simulink model "q3_3_2"  (R2022a)
settings: Solver=FixedStepAuto  StartTime=0.0  StopTime=200.0  FixedStep=5e-3  RelTol=1e-3
settings Model: Creator=user  LastModifiedBy=user

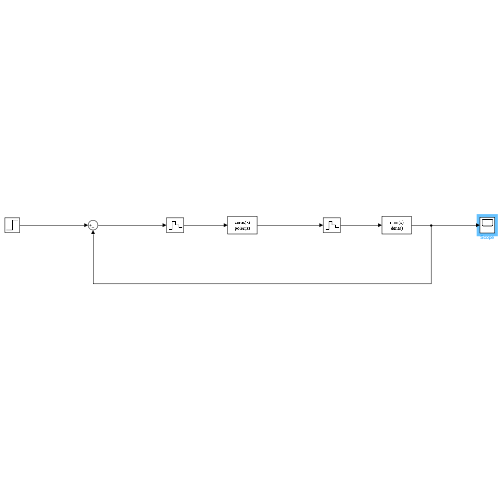
[thumbnail: Simulink's stored preview of the top-level diagram]
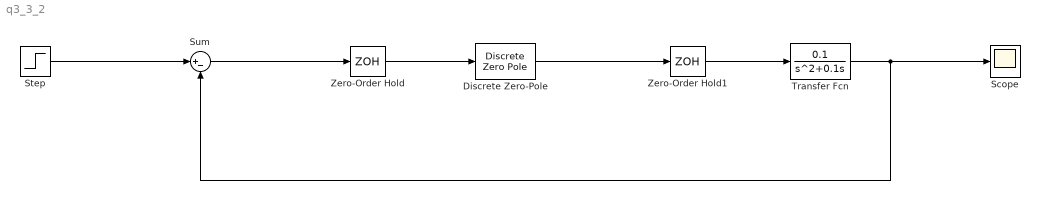
== system q3_3_2 ==
  Discrete Zero-Pole : DiscreteZeroPole  Zeros=[0.8]  Poles=[-0.8]  Gain=9  SampleTime=-1
  Scope : Scope
  Step : Step  SampleTime=0
  Sum : Sum  Inputs=|+-
  Transfer Fcn : TransferFcn  Numerator=[0.1]  Denominator=[1 0.1 0]
  Zero-Order Hold : ZeroOrderHold  SampleTime=-1
  Zero-Order Hold1 : ZeroOrderHold  SampleTime=-1
  wires:
  Step/1 -> Sum/1
  Discrete Zero-Pole/1 -> Zero-Order Hold1/1
  Zero-Order Hold/1 -> Discrete Zero-Pole/1
  Sum/1 -> Zero-Order Hold/1
  Zero-Order Hold1/1 -> Transfer Fcn/1
  Transfer Fcn/1 -> Sum/2, Scope/1
